simulink model "communicationExcavatorCAN_1"  (R2025a)
settings: Solver=VariableStepAuto  StartTime=0.0  StopTime=inf  RelTol=1e-3
undefined symbols (not defined in the file or in its folder): canChannel
libraries: canlib x6, canmsglib x4, aerolibanimutils x1
(part 2 of 2)

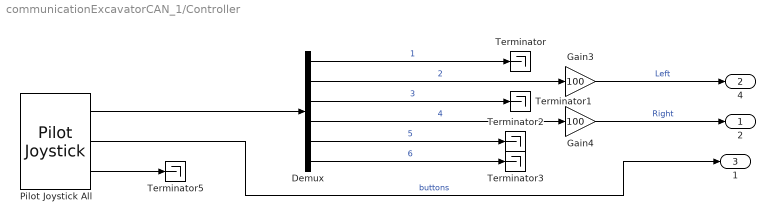
== system communicationExcavatorCAN_1/Controller ==
  Demux : Demux  Outputs=6
  Gain3 : Gain  Gain=100
  Gain4 : Gain  Gain=100
  Pilot Joystick All : aerolibanimutils/Pilot Joystick  JoystickID=Joystick2  OutputConfiguration=AllOutputs  SampleTime=1/50
      settings: LibrarySourceBlock=aerolibanimutils/Pilot Joystick All
  Terminator{,1..3,5} (5 alike) : Terminator
  2 : Outport
  4 : Outport  Port=2
  1 : Outport  Port=3
  wires:
  Demux/6 -> Terminator3/1  "6"
  Demux/5 -> Terminator2/1  "5"
  Pilot Joystick All/3 -> Terminator5/1
  Pilot Joystick All/1 -> Demux/1
  Demux/1 -> Terminator/1  "1"
  Demux/4 -> Gain4/1  "4"
  Pilot Joystick All/2 -> 1/1  "buttons"
  Demux/3 -> Terminator1/1  "3"
  Demux/2 -> Gain3/1  "2"
  Gain3/1 -> 4/1  "Left"
  Gain4/1 -> 2/1  "Right"

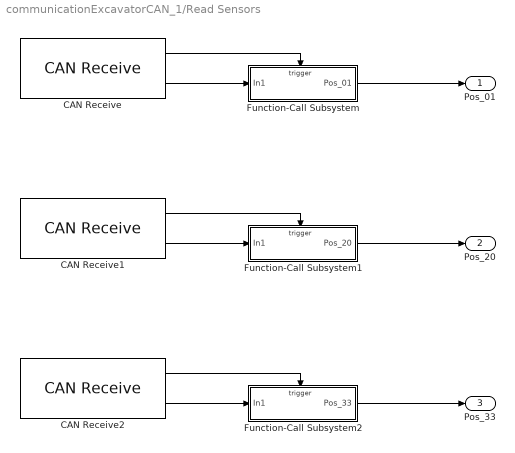
== system communicationExcavatorCAN_1/Read Sensors ==
  CAN Receive : canlib/CAN Receive  BlockHandle=626.0001  Device=Kvaser USBcan Light 1 (Channel 1)  DeviceMenu=Kvaser USBcan Light 1 (Channel 1)  ObjConstructor=canChannel('Kvaser', 'USBcan Light 1', 1)  EnableStandardIDsFilter=off  StdIDsCombo=Allow all  StandardIDs=0  EnableExtendedIDsFilter=off  ExtIDsCombo=Allow all  ExtendedIDs=0  SampleTime=0.01  MsgsPerTimestep=all  InternalFilterUpdateStatus=on  BusOutput=off
  CAN Receive1 : canlib/CAN Receive  BlockHandle=629.0001  Device=Kvaser USBcan Light 1 (Channel 1)  DeviceMenu=Kvaser USBcan Light 1 (Channel 1)  ObjConstructor=canChannel('Kvaser', 'USBcan Light 1', 1)  EnableStandardIDsFilter=off  StdIDsCombo=Allow all  StandardIDs=0  EnableExtendedIDsFilter=off  ExtIDsCombo=Allow all  ExtendedIDs=0  SampleTime=0.01  MsgsPerTimestep=all  InternalFilterUpdateStatus=on  BusOutput=off
  CAN Receive2 : canlib/CAN Receive  BlockHandle=632.0001  Device=Kvaser USBcan Light 1 (Channel 1)  DeviceMenu=Kvaser USBcan Light 1 (Channel 1)  ObjConstructor=canChannel('Kvaser', 'USBcan Light 1', 1)  EnableStandardIDsFilter=off  StdIDsCombo=Allow all  StandardIDs=0  EnableExtendedIDsFilter=off  ExtIDsCombo=Allow all  ExtendedIDs=0  SampleTime=0.01  MsgsPerTimestep=all  InternalFilterUpdateStatus=on  BusOutput=off
  Function-Call Subsystem : Subsystem  TreatAsAtomicUnit=on
  Function-Call Subsystem1 : Subsystem  TreatAsAtomicUnit=on
  Function-Call Subsystem2 : Subsystem  TreatAsAtomicUnit=on
  Pos_01 : Outport
  Pos_20 : Outport  Port=2
  Pos_33 : Outport  Port=3
  wires:
  CAN Receive/2 -> Function-Call Subsystem/1(In1)
  CAN Receive1/2 -> Function-Call Subsystem1/1(In1)
  CAN Receive/1 -> Function-Call Subsystem/Trigger
  CAN Receive2/2 -> Function-Call Subsystem2/1(In1)
  Function-Call Subsystem2/1(Pos_33) -> Pos_33/1
  Function-Call Subsystem/1(Pos_01) -> Pos_01/1
  CAN Receive2/1 -> Function-Call Subsystem2/Trigger
  CAN Receive1/1 -> Function-Call Subsystem1/Trigger
  Function-Call Subsystem1/1(Pos_20) -> Pos_20/1

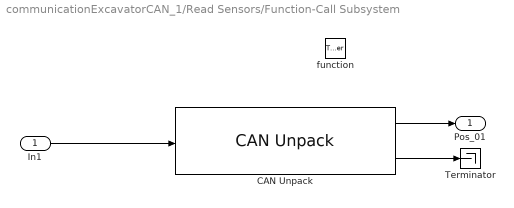
== system communicationExcavatorCAN_1/Read Sensors/Function-Call Subsystem ==
  In1 : Inport
  function : TriggerPort  TriggerType=function-call  VariantControl=(inherit)
  CAN Unpack : canmsglib/CAN Unpack  CANdbFile=C:\Users\Viktor Traktor\Downloads\VolvoExcavator\systemIdentificationVolvo\ec20_kth.dbc  MsgList=Rot_01  MsgName=Rot_01  MsgIDType=Extended (29-bit identifier)  MsgIdentifier=419408385  MsgLength=8  SignalInfo={'SnsrPos_01','0','32','LE','unsigned','Standard','0','1','0','0','4294967295';'SnsrRPM_01','32','16','LE','unsigned','Standard','0','1','0','0','65535'}  IDPort=off  TimestampPort=off  ErrorPort=off  RemotePort=off  LengthPort=off  StatusPort=off  ApplyMinMax=off
      settings: LibrarySourceBlock=canlib/CAN Unpack  DataFormat=CANdb specified signals
  Terminator : Terminator
  Pos_01 : Outport
  wires:
  In1/1 -> CAN Unpack/1
  CAN Unpack/1 -> Pos_01/1
  CAN Unpack/2 -> Terminator/1

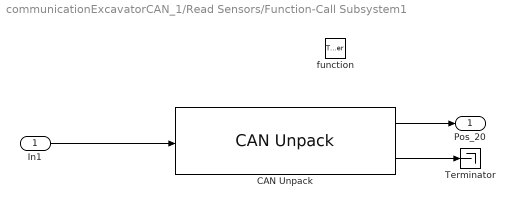
== system communicationExcavatorCAN_1/Read Sensors/Function-Call Subsystem1 ==
  In1 : Inport
  function : TriggerPort  TriggerType=function-call  VariantControl=(inherit)
  CAN Unpack : canmsglib/CAN Unpack  CANdbFile=C:\Users\Viktor Traktor\Downloads\VolvoExcavator\systemIdentificationVolvo\ec20_kth.dbc  MsgList=Rot_20  MsgName=Rot_20  MsgIDType=Extended (29-bit identifier)  MsgIdentifier=419408416  MsgLength=8  SignalInfo={'SnsrPos_20','0','32','LE','unsigned','Standard','0','1','0','0','4294967295';'SnsrRPM_20','32','16','LE','unsigned','Standard','0','1','0','0','65535'}  IDPort=off  TimestampPort=off  ErrorPort=off  RemotePort=off  LengthPort=off  StatusPort=off  ApplyMinMax=off
      settings: LibrarySourceBlock=canlib/CAN Unpack  DataFormat=CANdb specified signals
  Terminator : Terminator
  Pos_20 : Outport
  wires:
  CAN Unpack/1 -> Pos_20/1
  In1/1 -> CAN Unpack/1
  CAN Unpack/2 -> Terminator/1

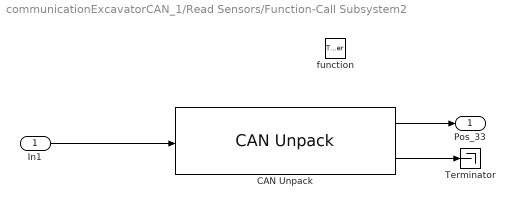
== system communicationExcavatorCAN_1/Read Sensors/Function-Call Subsystem2 ==
  In1 : Inport
  function : TriggerPort  TriggerType=function-call  VariantControl=(inherit)
  CAN Unpack : canmsglib/CAN Unpack  CANdbFile=C:\Users\Viktor Traktor\Downloads\VolvoExcavator\systemIdentificationVolvo\ec20_kth.dbc  MsgList=Rot_33  MsgName=Rot_33  MsgIDType=Extended (29-bit identifier)  MsgIdentifier=419408435  MsgLength=8  SignalInfo={'SnsrPos_33','0','32','LE','unsigned','Standard','0','1','0','0','4294967295';'SnsrRPM_33','32','16','LE','unsigned','Standard','0','1','0','0','65535'}  IDPort=off  TimestampPort=off  ErrorPort=off  RemotePort=off  LengthPort=off  StatusPort=off  ApplyMinMax=off
      settings: LibrarySourceBlock=canlib/CAN Unpack  DataFormat=CANdb specified signals
  Terminator : Terminator
  Pos_33 : Outport
  wires:
  In1/1 -> CAN Unpack/1
  CAN Unpack/1 -> Pos_33/1
  CAN Unpack/2 -> Terminator/1
